simulink model "GaitAlgorithm_arduino_V4_2024b"  (R2024b)
settings: Solver=FixedStepAuto  StartTime=0.0  StopTime=inf  RelTol=1e-3  EnableMultiTasking=on
undefined symbols (not defined in the file): f
libraries: arduinolib x2, instrumentlib x1
settings Model: ExtModeTrigDuration=2  Creator=82108  LastModifiedBy=admin
settings SolverCC: AutoInsertRateTranBlk=on
settings OptimizationCC: EnhancedBackFolding=on  PassReuseOutputArgsAs=Individual arguments  ZeroExternalMemoryAtStartup=off  ZeroInternalMemoryAtStartup=off  MaxStackSize=64  OptimizeBlockOrder=speed  DifferentSizesBufferReuse=on  OptimizationCustomize=off  EfficientTunableParamExpr=on
settings DebuggingCC: ParameterTunabilityLossMsg=error
settings HardwareCC: ProdBitPerInt=16  ProdBitPerPointer=16  ProdBitPerSizeT=16  ProdBitPerPtrDiffT=16  ProdLargestAtomicFloat=None  ProdWordSize=8  ProdHWDeviceType=Atmel->AVR  TargetBitPerPointer=64  TargetBitPerSizeT=64  TargetBitPerPtrDiffT=64  TargetLongLongMode=on  TargetIntDivRoundTo=Zero  TargetEndianess=LittleEndian  TargetWordSize=64  TargetHWDeviceType=Custom Processor->MATLAB Host Computer  ProdEqTarget=off
settings SFSimCC: MATLABDynamicMemAlloc=off
settings RTWCC: Description=Embedded Coder  SystemTargetFile=ert.tlc  HardwareBoard=Arduino Uno  TemplateMakefile=ert_default_tmf  Toolchain=Arduino AVR  BuildConfiguration=Faster Runs  GPUComputeCapability=3.5
settings CodeAppCC: ForceParamTrailComments=on  IgnoreCustomStorageClasses=off  OperatorAnnotations=on  SimulinkDataObjDesc=on  SFDataObjDesc=on  InsertBlockDesc=on
settings ERTTargetCC: SupportContinuousTime=on  SupportVariableSizeSignals=on  ExtModeTransport=3  ExtModeStaticAlloc=on  ExtModeAutomaticAllocSize=off  ExtModeStaticAllocSize=250  ExtModeMexFile=ext_xcp  ExtModeIntrfLevel=Level2 - Open  InlinedParameterPlacement=Hierarchical  DynamicArrayContainerType=coder::array

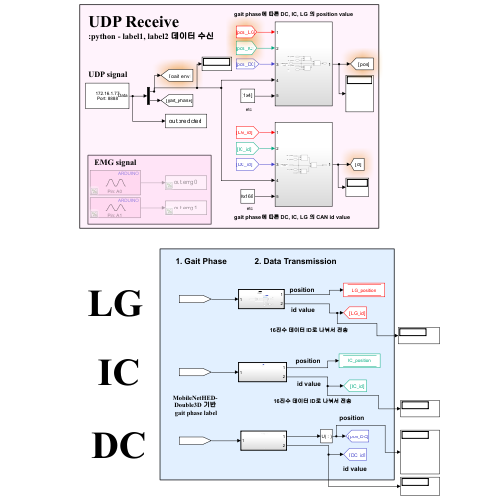
[thumbnail: Simulink's stored preview of the top-level diagram]
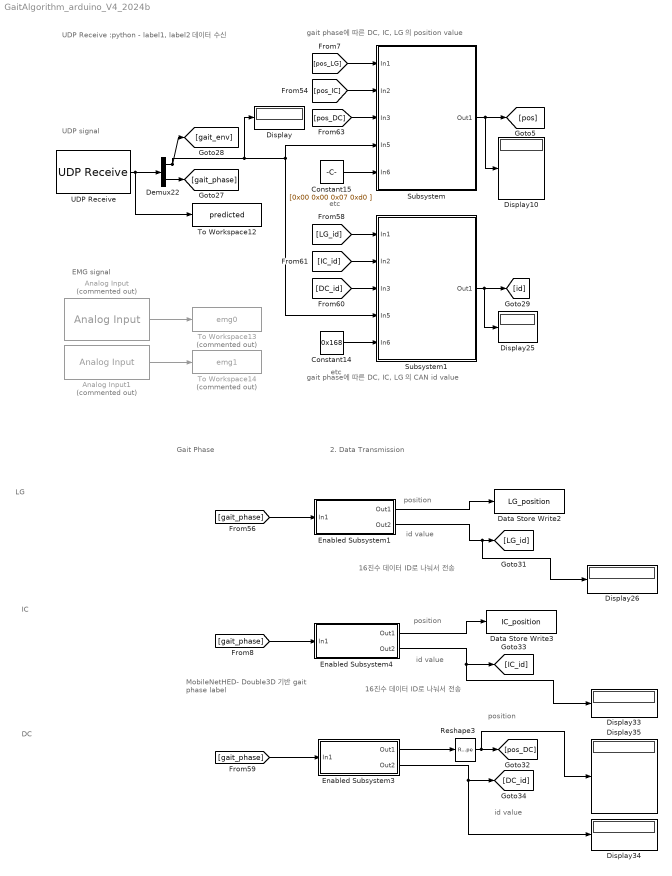
== system GaitAlgorithm_arduino_V4_2024b ==
  note: gait phase에 따른 DC, IC, LG 의 position value
  note: position
  note: DC
  note: MobileNetHED- Double3D 기반
      | gait phase label
  note: 16진수 데이터 ID로 나눠서 전송
  note: id value
  note: Gait Phase
  note: 2. Data Transmission
  note: 16진수 데이터 ID로 나눠서 전송
  note: id value
  note: position
  note: LG
  note: IC
  note: position
  note: id value
  note: gait phase에 따른 DC, IC, LG 의 CAN id value
  note: UDP signal
  note: EMG signal
  note: etc
  note: etc
  note: UDP Receive
      | :python - label1, label2 데이터 수신
  Analog Input : arduinolib/Analog Input  Commented=on  pinNumber=0  ReadResultsOnly=off  ConversionTriggerSource=Software  ExternalTriggerType=uint32( 0 )  OutputDataType=uint16  EnableConversionCompleteNotify=off  EnableOuputStatus=off  SampleTime=0.01  blockPlatform=arduino
      settings: SourceProductName=Common
  Analog Input1 : arduinolib/Analog Input  Commented=on  pinNumber=1  ReadResultsOnly=off  ConversionTriggerSource=Software  ExternalTriggerType=uint32( 0 )  OutputDataType=uint16  EnableConversionCompleteNotify=off  EnableOuputStatus=off  SampleTime=0.01  blockPlatform=arduino
      settings: SourceProductName=Common
  Constant14 : Constant  Value=0x168  OutDataTypeStr=uint16
  Constant15 : Constant  Value=[0x00 0x00 0x07 0xd0 ]  OutDataTypeStr=uint16
  Data Store Write2 : DataStoreWrite  DataStoreName=LG_position  IndexOptions=Index vector (dialog)  Indices=1  OutputSizes=1
  Data Store Write3 : DataStoreWrite  DataStoreName=IC_position  IndexOptions=Index vector (dialog)  Indices=1  OutputSizes=1
  Demux22 : Demux  Outputs=2
  Display{,10,25..26,33..35} (7 alike) : Display
  Enabled Subsystem1 : Subsystem  TreatAsAtomicUnit=on
  Enabled Subsystem3 : Subsystem  TreatAsAtomicUnit=on
  Enabled Subsystem4 : Subsystem  TreatAsAtomicUnit=on
  Reshape3 : Reshape
  Subsystem : Subsystem
  Subsystem1 : Subsystem
  To Workspace12 : ToWorkspace  VariableName=predicted  SaveFormat=Timeseries  SampleTime=-1
  To Workspace13 : ToWorkspace  Commented=on  VariableName=emg0  SaveFormat=Timeseries  SampleTime=-1
  To Workspace14 : ToWorkspace  Commented=on  VariableName=emg1  SaveFormat=Timeseries  SampleTime=-1
  UDP Receive : instrumentlib/UDP Receive  LocalAddress=172.16.1.77  LocalPort=8888  EnablePortSharing=off  Host=localhost  Port=9090  GetLatestData=off  DataSize=[ 2, 1 ]  DataType=uint8  ASCIIFormatting=%f,  Terminator=LF  CustomTerminator=10  ByteOrder=big-endian  EnableBlockingMode=on  Timeout=10  SampleTime=0.1  SimulateUsing=Interpreted execution
  wires:
  Enabled Subsystem4/2(Out2) -> Display33/1, [IC_id]
  Enabled Subsystem4/1(Out1) -> Data Store Write3/1
  Enabled Subsystem3/1(Out1) -> Reshape3/1
  Enabled Subsystem3/2(Out2) -> Display34/1, [DC_id]
  [pos_IC] -> Subsystem/2(In2)
  [IC_id] -> Subsystem1/2(In2)
  Constant15/1 -> Subsystem/5(In6)
  Constant14/1 -> Subsystem1/5(In6)
  Subsystem/1(Out1) -> Display10/1, [pos]
  Subsystem1/1(Out1) -> Display25/1, [id]
  Reshape3/1 -> Display35/1, [pos_DC]
  Enabled Subsystem1/2(Out2) -> Display26/1, [LG_id]
  Enabled Subsystem1/1(Out1) -> Data Store Write2/1
  Analog Input/1 -> To Workspace13/1
  Analog Input1/1 -> To Workspace14/1
  UDP Receive/1 -> Demux22/1, To Workspace12/1
  [gait_phase] -> Enabled Subsystem1/1(In1)
  [gait_phase] -> Enabled Subsystem4/1(In1)
  [gait_phase] -> Enabled Subsystem3/1(In1)
  Demux22/2 -> [gait_phase]
  Demux22/1 -> Display/1, Subsystem1/4(In5), Subsystem/4(In5), [gait_env]
  [pos_LG] -> Subsystem/1(In1)
  [pos_DC] -> Subsystem/3(In3)
  [DC_id] -> Subsystem1/3(In3)
  [LG_id] -> Subsystem1/1(In1)

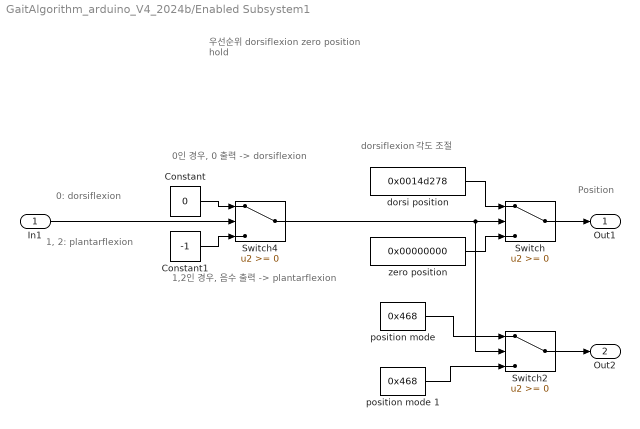
== system GaitAlgorithm_arduino_V4_2024b/Enabled Subsystem1 ==
  note: dorsiflexion 각도 조절
  note: 우선순위
      | dorsiflexion
      | zero position
      | hold
  note: Position
  note: 0: dorsiflexion
  note: 1, 2: plantarflexion
  note: 1,2인 경우, 음수 출력 -> plantarflexion
  note: 0인 경우, 0 출력 -> dorsiflexion
  In1 : Inport
  Constant : Constant  Value=0
  Constant1 : Constant  Value=-1
  Switch : Switch  OutDataTypeStr=uint32  SaturateOnIntegerOverflow=off  InputSameDT=off
  Switch2 : Switch  OutDataTypeStr=uint32  SaturateOnIntegerOverflow=off  InputSameDT=off
  Switch4 : Switch  SaturateOnIntegerOverflow=off  InputSameDT=off
  dorsi position : Constant  Value=0x0014d278
  "position mode " : Constant  Value=0x468
  position mode 1 : Constant  Value=0x468
  zero position : Constant  Value=0x00000000
  Out1 : Outport
  Out2 : Outport  Port=2
  wires:
  Switch/1 -> Out1/1
  dorsi position/1 -> Switch/1
  "position mode "/1 -> Switch2/1
  In1/1 -> Switch4/2
  Constant/1 -> Switch4/1
  Constant1/1 -> Switch4/3
  zero position/1 -> Switch/3
  Switch2/1 -> Out2/1
  position mode 1/1 -> Switch2/3
  Switch4/1 -> Switch2/2, Switch/2

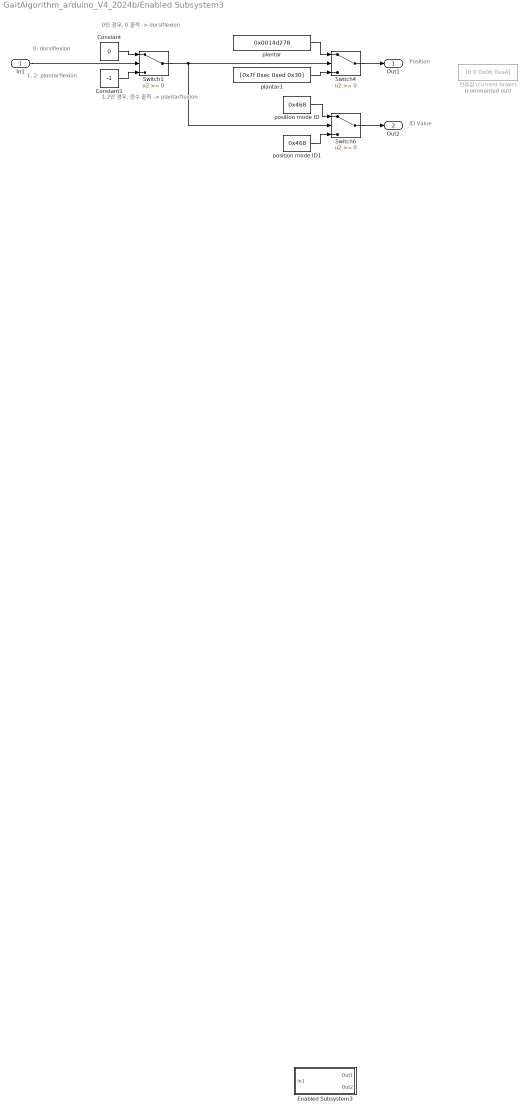
== system GaitAlgorithm_arduino_V4_2024b/Enabled Subsystem3 ==
  note: ID Value
  note: Position
  note: 1,2인 경우, 음수 출력 -> plantarflexion
  note: 0인 경우, 0 출력 -> dorsiflexion
  note: 1, 2: plantarflexion
  note: 0: dorsiflexion
  In1 : Inport
  Constant : Constant  Value=0
  Constant1 : Constant  Value=-1
  Enabled Subsystem3 : Subsystem  TreatAsAtomicUnit=on
  Switch1 : Switch  SaturateOnIntegerOverflow=off  InputSameDT=off
  Switch4 : Switch  OutDataTypeStr=uint32  SaturateOnIntegerOverflow=off  InputSameDT=off
  Switch6 : Switch  OutDataTypeStr=uint32  SaturateOnIntegerOverflow=off  InputSameDT=off
  plantar : Constant  Value=0x0014d278
  plantar1 : Constant  Value=[0x7f 0xec 0xed 0x30]
  position mode ID : Constant  Value=0x468
  position mode ID1 : Constant  Value=0x468
  전류값 (current brake) : Constant  Commented=on  Value=[0 0 0x06 0xa4]  OutDataTypeStr=uint8
  Out1 : Outport
  Out2 : Outport  Port=2
  wires:
  Switch6/1 -> Out2/1
  plantar/1 -> Switch4/1
  position mode ID/1 -> Switch6/1
  position mode ID1/1 -> Switch6/3
  Switch4/1 -> Out1/1
  In1/1 -> Switch1/2
  Constant/1 -> Switch1/1
  Constant1/1 -> Switch1/3
  Switch1/1 -> Switch6/2, Switch4/2
  plantar1/1 -> Switch4/3

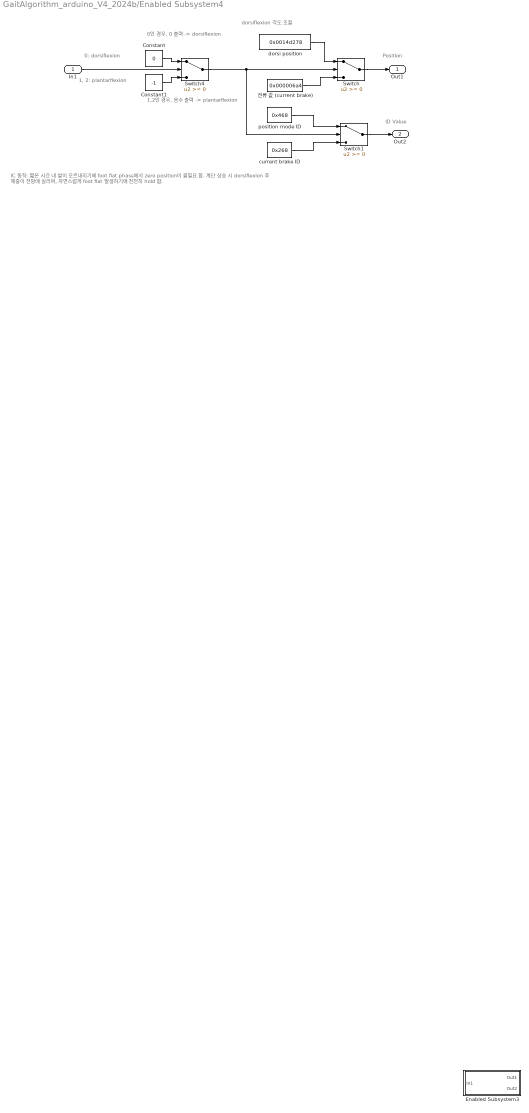
== system GaitAlgorithm_arduino_V4_2024b/Enabled Subsystem4 ==
  note: ID Value
  note: Position
  note: dorsiflexion 각도 조절
  note: IC 동작: 짧은 시간 내 발이 오르내리기에 foot flat phase에서 zero position이 불필요 함.
      | 계단 상승 시 dorsiflexion 후 체중이 전방에 실리며, 자연스럽게 foot flat 발생하기에 천천히 hold 함.
  note: 1,2인 경우, 음수 출력 -> plantarflexion
  note: 0인 경우, 0 출력 -> dorsiflexion
  note: 1, 2: plantarflexion
  note: 0: dorsiflexion
  In1 : Inport
  " 전류 값 (current brake)" : Constant  Value=0x000006a4
  Constant : Constant  Value=0
  Constant1 : Constant  Value=-1
  Enabled Subsystem3 : Subsystem  TreatAsAtomicUnit=on
  Switch : Switch  OutDataTypeStr=uint32  SaturateOnIntegerOverflow=off  InputSameDT=off
  Switch1 : Switch  OutDataTypeStr=uint32  SaturateOnIntegerOverflow=off  InputSameDT=off
  Switch4 : Switch  SaturateOnIntegerOverflow=off  InputSameDT=off
  current brake ID : Constant  Value=0x268
  dorsi position : Constant  Value=0x0014d278
  position mode ID : Constant  Value=0x468
  Out1 : Outport
  Out2 : Outport  Port=2
  wires:
  Switch/1 -> Out1/1
  Switch1/1 -> Out2/1
  dorsi position/1 -> Switch/1
  " 전류 값 (current brake)"/1 -> Switch/3
  position mode ID/1 -> Switch1/1
  current brake ID/1 -> Switch1/3
  In1/1 -> Switch4/2
  Constant/1 -> Switch4/1
  Switch4/1 -> Switch1/2, Switch/2
  Constant1/1 -> Switch4/3

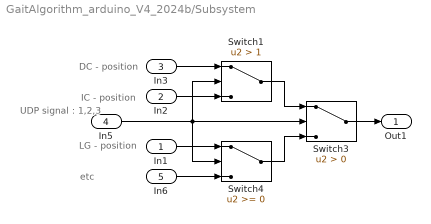
== system GaitAlgorithm_arduino_V4_2024b/Subsystem ==
  note: UDP signal
      | : 1,2,3
  note: LG - position
  note: IC - position
  note: DC - position
  note: etc
  In1 : Inport
  In2 : Inport  Port=2
  In3 : Inport  Port=3
  In5 : Inport  Port=4
  In6 : Inport  Port=5
  Switch1 : Switch  Criteria=u2 > Threshold  Threshold=1  SaturateOnIntegerOverflow=off  InputSameDT=off
  Switch3 : Switch  Criteria=u2 > Threshold  SaturateOnIntegerOverflow=off  InputSameDT=off
  Switch4 : Switch  SaturateOnIntegerOverflow=off  InputSameDT=off
  Out1 : Outport
  wires:
  In2/1 -> Switch1/3
  In3/1 -> Switch1/1
  Switch1/1 -> Switch3/1
  Switch3/1 -> Out1/1
  In5/1 -> Switch4/2, Switch3/2, Switch1/2
  Switch4/1 -> Switch3/3
  In1/1 -> Switch4/1
  In6/1 -> Switch4/3

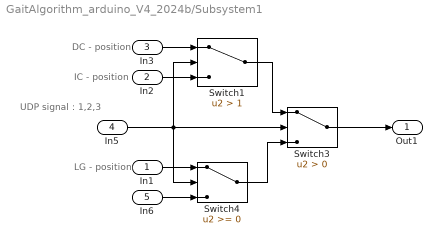
== system GaitAlgorithm_arduino_V4_2024b/Subsystem1 ==
  note: LG - position
  note: DC - position
  note: UDP signal
      | : 1,2,3
  note: IC - position
  In1 : Inport
  In2 : Inport  Port=2
  In3 : Inport  Port=3
  In5 : Inport  Port=4
  In6 : Inport  Port=5
  Switch1 : Switch  Criteria=u2 > Threshold  Threshold=1  SaturateOnIntegerOverflow=off  InputSameDT=off
  Switch3 : Switch  Criteria=u2 > Threshold  SaturateOnIntegerOverflow=off  InputSameDT=off
  Switch4 : Switch  SaturateOnIntegerOverflow=off  InputSameDT=off
  Out1 : Outport
  wires:
  In2/1 -> Switch1/3
  In3/1 -> Switch1/1
  Switch1/1 -> Switch3/1
  Switch3/1 -> Out1/1
  In5/1 -> Switch1/2, Switch3/2, Switch4/2
  Switch4/1 -> Switch3/3
  In1/1 -> Switch4/1
  In6/1 -> Switch4/3

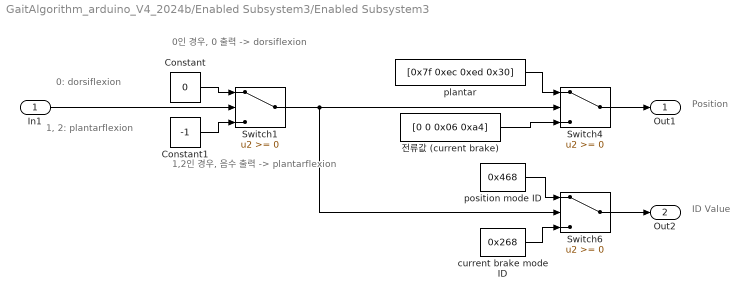
== system GaitAlgorithm_arduino_V4_2024b/Enabled Subsystem3/Enabled Subsystem3 ==
  note: ID Value
  note: Position
  note: 1,2인 경우, 음수 출력 -> plantarflexion
  note: 0인 경우, 0 출력 -> dorsiflexion
  note: 1, 2: plantarflexion
  note: 0: dorsiflexion
  In1 : Inport
  Constant : Constant  Value=0
  Constant1 : Constant  Value=-1
  Switch1 : Switch  SaturateOnIntegerOverflow=off  InputSameDT=off
  Switch4 : Switch  OutDataTypeStr=uint32  SaturateOnIntegerOverflow=off  InputSameDT=off
  Switch6 : Switch  OutDataTypeStr=uint32  SaturateOnIntegerOverflow=off  InputSameDT=off
  current brake mode ID : Constant  Value=0x268
  plantar : Constant  Value=[0x7f 0xec 0xed 0x30]
  position mode ID : Constant  Value=0x468
  전류값 (current brake) : Constant  Value=[0 0 0x06 0xa4]  OutDataTypeStr=uint8
  Out1 : Outport
  Out2 : Outport  Port=2
  wires:
  Switch6/1 -> Out2/1
  plantar/1 -> Switch4/1
  전류값 (current brake)/1 -> Switch4/3
  position mode ID/1 -> Switch6/1
  current brake mode ID/1 -> Switch6/3
  Switch4/1 -> Out1/1
  In1/1 -> Switch1/2
  Constant/1 -> Switch1/1
  Constant1/1 -> Switch1/3
  Switch1/1 -> Switch6/2, Switch4/2

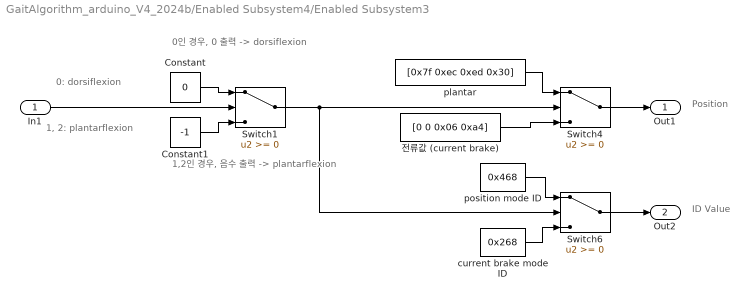
== system GaitAlgorithm_arduino_V4_2024b/Enabled Subsystem4/Enabled Subsystem3 ==
  note: ID Value
  note: Position
  note: 1,2인 경우, 음수 출력 -> plantarflexion
  note: 0인 경우, 0 출력 -> dorsiflexion
  note: 1, 2: plantarflexion
  note: 0: dorsiflexion
  In1 : Inport
  Constant : Constant  Value=0
  Constant1 : Constant  Value=-1
  Switch1 : Switch  SaturateOnIntegerOverflow=off  InputSameDT=off
  Switch4 : Switch  OutDataTypeStr=uint32  SaturateOnIntegerOverflow=off  InputSameDT=off
  Switch6 : Switch  OutDataTypeStr=uint32  SaturateOnIntegerOverflow=off  InputSameDT=off
  current brake mode ID : Constant  Value=0x268
  plantar : Constant  Value=[0x7f 0xec 0xed 0x30]
  position mode ID : Constant  Value=0x468
  전류값 (current brake) : Constant  Value=[0 0 0x06 0xa4]  OutDataTypeStr=uint8
  Out1 : Outport
  Out2 : Outport  Port=2
  wires:
  Switch6/1 -> Out2/1
  plantar/1 -> Switch4/1
  전류값 (current brake)/1 -> Switch4/3
  position mode ID/1 -> Switch6/1
  current brake mode ID/1 -> Switch6/3
  Switch4/1 -> Out1/1
  In1/1 -> Switch1/2
  Constant/1 -> Switch1/1
  Constant1/1 -> Switch1/3
  Switch1/1 -> Switch6/2, Switch4/2
